simulink model "simu_state_space_model"  (R2015a)
settings: Solver=ode3  StartTime=0.0  StopTime=100  FixedStep=0.001  RelTol=1e-3
undefined symbols (not defined in the file or in its folder): A, B, C, D
undefined symbols (not defined in the file): A2, B2, C2, D2
libraries: simulink x2
settings Model: Creator=Xiaotian  LastModifiedBy=Xiaotian

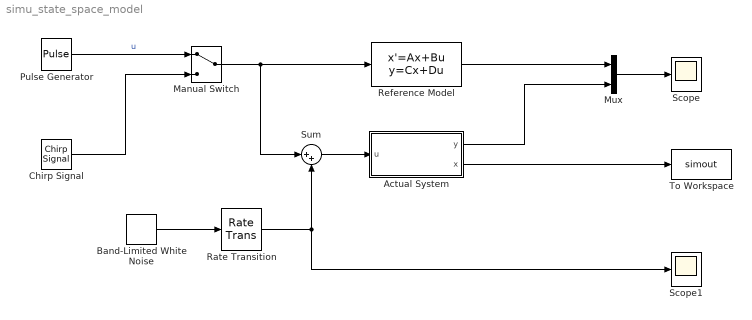
== system simu_state_space_model ==
  Actual System : Subsystem  mask{A=A2, B=B2, C=C2, D=D2}
  Band-Limited White Noise : simulink/Sources/Band-Limited White Noise  Cov=[0.0001]  Ts=0.1  seed=[23341]
  Chirp Signal : simulink/Sources/Chirp Signal  f1=0.1  T=100  f2=1
  Manual Switch : ManualSwitch
  Mux : Mux  Inputs=2
  Pulse Generator : DiscretePulseGenerator  PulseType=Time based  Period=30  PulseWidth=50
  Rate Transition : RateTransition
  Reference Model : StateSpace  A=A  B=B  C=C  D=D  X0=0
  Scope : Scope
  Scope1 : Scope
  Sum : Sum  Inputs=|++
  To Workspace : ToWorkspace  VariableName=simout  SaveFormat=Timeseries  SampleTime=-1
  wires:
  Mux/1 -> Scope/1
  Reference Model/1 -> Mux/1
  Actual System/1(y) -> Mux/2
  Actual System/2(x) -> To Workspace/1
  Manual Switch/1 -> Sum/1, Reference Model/1
  Pulse Generator/1 -> Manual Switch/1  "u"
  Chirp Signal/1 -> Manual Switch/2
  Sum/1 -> Actual System/1(u)
  Band-Limited White Noise/1 -> Rate Transition/1
  Rate Transition/1 -> Scope1/1, Sum/2

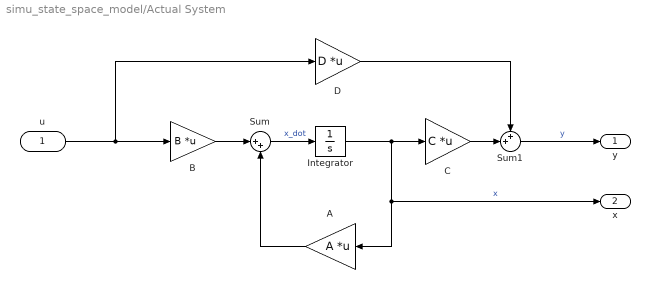
== system simu_state_space_model/Actual System ==
  u : Inport
  A : Gain  Gain=A  Multiplication=Matrix(K*u)
  B : Gain  Gain=B  Multiplication=Matrix(K*u)
  C : Gain  Gain=C  Multiplication=Matrix(K*u)
  D : Gain  Gain=D  Multiplication=Matrix(K*u)
  Integrator : Integrator
  Sum : Sum  Inputs=|++
  Sum1 : Sum  Inputs=++|
  y : Outport
  x : Outport  Port=2
  wires:
  B/1 -> Sum/1
  Sum/1 -> Integrator/1  "x_dot"
  A/1 -> Sum/2
  u/1 -> D/1, B/1
  Sum1/1 -> y/1  "y"
  D/1 -> Sum1/1
  Integrator/1 -> x/1, A/1, C/1  "x"
  C/1 -> Sum1/2
